simulink model "controlMCUSlugsMKII"  (Simulink 6.6)
settings: Solver=FixedStepDiscrete  StartTime=0.0  StopTime=10.0  FixedStep=0.01  RelTol=1e-3
InitFcn:
  | mcuInit
values from neighbouring files (symbols this model uses):
  T = 0.01    [initGPS.m]    (also in mcuInit.m)
undefined symbols (not defined in the file or in its folder): apSampleTime, bankCommandLimit, baseHeight, bda, bde, bdr, bdt, bICda, bICde, bICdr, bICdt, controlMCUInit, daLimit, deLimit, drLimit, dtLimit, getAccBias, getAccels, getAttitude, getMidLevelCommands, getPassValues, getPidIdx, getWP, getXYZ, gsRead, ISA_g, mda, mde, mdr, mdt, mICda, mICde, mICdr, mICdt, pitchCommandLimit, prepareTelemetry, protParseDecode, protParseDecodeGS, readIpc, send2GS, setCurrentCommands, setDiagnosticFloat, setDiagnosticShort, setNavLat, setNavLong, setNavNav, u1, u2, updateEuler, updateLoad, updatePQR, updatePWM, updatePWM2, y1
libraries: dsPICdrivers x82, simulink x43, SLUGS_Library x27, aerolibconvert2 x3, aerolibutil x3
(part 3 of 5)

== system controlMCUSlugsMKII/Trim Vals/Grab I.C./Convert to Rad2 ==
  IC : Inport  Orientation=down
  Add : Sum  OutScaling=2^-10
  Constant1 : Constant  Value=slopem
  Constant2 : Constant  Value=interceptb
  Data Type Conversion : DataTypeConversion  OutDataTypeMode=single
  Divide : Product  OutScaling=2^-10
  Angle (rad) : Outport
  wires:
  Data Type Conversion/1 -> Angle (rad)/1
  IC/1 -> Divide/1
  Constant2/1 -> Add/2
  Divide/1 -> Add/1
  Add/1 -> Data Type Conversion/1
  Constant1/1 -> Divide/2

== system controlMCUSlugsMKII/Trim Vals/Grab I.C./Convert to Rad3 ==
  IC : Inport  Orientation=down
  Add : Sum  OutScaling=2^-10
  Constant1 : Constant  Value=slopem
  Constant2 : Constant  Value=interceptb
  Data Type Conversion : DataTypeConversion  OutDataTypeMode=single
  Divide : Product  OutScaling=2^-10
  Angle (rad) : Outport
  wires:
  Constant1/1 -> Divide/2
  Add/1 -> Data Type Conversion/1
  Divide/1 -> Add/1
  Constant2/1 -> Add/2
  IC/1 -> Divide/1
  Data Type Conversion/1 -> Angle (rad)/1

== system controlMCUSlugsMKII/Trim Vals/Log  Trims Using PWM High [groundStationDriver.c]/Report Airspeed ==
  Um : Inport  Orientation=down
  Data Type Conversion4 : DataTypeConversion  OutDataTypeMode=uint16  SampleTime=apSampleTime  SaturateOnIntegerOverflow=on
  Gain4 : Gain  Gain=1000
  Update PWM  Commands4 : dsPICdrivers/OTHERS/C Function Call  Tag=dsPIC_dsPIC_CFunctionCall  fctName='updatePWM2'  INPUT_SIZE=1  INPUT1=uint16  INPUT2=uint8  INPUT3=--  OUTPUT_SIZE=1  OUTPUT1=--  SampleTime=-1  InputType=[ 4 2 ]  OutputType=[ ]  FctDeclaration=extern void updatePWM2(uint16_T u1, uint8_T u2);  FctCall=updatePWM2(%u1, %u2);  OrderingInOutPopup=None
  dlf1 : Constant  Value=4  OutDataTypeMode=uint8
  wires:
  Data Type Conversion4/1 -> Update PWM  Commands4/1
  dlf1/1 -> Update PWM  Commands4/2
  Gain4/1 -> Data Type Conversion4/1
  Um/1 -> Gain4/1

== system controlMCUSlugsMKII/Update PWM Commands and Send Telemetry/Generate PWM Signals Based on the Control Type/If  Control Type Is Manual ==
  Pilot (IC) : Inport
  Action Port : ActionPort  ActionType=then
  Demux : Demux
  Gain{,1..3} (4 alike) : Gain  Gain=0.5
  myMux Fun1 : Stateflow chart
  PWM : Outport
  wires:
  Gain/1 -> myMux Fun1/1(u1)
  Gain1/1 -> myMux Fun1/2(u2)
  Gain2/1 -> myMux Fun1/3(u3)
  Gain3/1 -> myMux Fun1/4(u4)
  Demux/1 -> Gain/1
  Demux/2 -> Gain1/1
  Demux/3 -> Gain2/1
  Demux/4 -> Gain3/1
  myMux Fun1/1(y) -> PWM/1
  Pilot (IC)/1 -> Demux/1

== system controlMCUSlugsMKII/Update PWM Commands and Send Telemetry/Generate PWM Signals Based on the Control Type/If  Control Type Is Passthrough ==
  Pilot (IC) : Inport
  Action Port : ActionPort  ActionType=elseif
  Demux : Demux
  Gain{,1..3} (4 alike) : Gain  Gain=0.5
  myMux Fun1 : Stateflow chart
  PWM (abs) : Outport
  wires:
  Gain/1 -> myMux Fun1/1(u1)
  Gain1/1 -> myMux Fun1/2(u2)
  Gain2/1 -> myMux Fun1/3(u3)
  Gain3/1 -> myMux Fun1/4(u4)
  Demux/1 -> Gain/1
  Demux/2 -> Gain1/1
  Demux/3 -> Gain2/1
  Demux/4 -> Gain3/1
  myMux Fun1/1(y) -> PWM (abs)/1
  Pilot (IC)/1 -> Demux/1

== system controlMCUSlugsMKII/Update PWM Commands and Send Telemetry/Generate PWM Signals Based on the Control Type/If  Control Type Is Selective Passthrough ==
  PWM(rad) : Inport
  Pilot (IC) : Inport  Port=2
  Action Port : ActionPort  ActionType=elseif
  Convert to PWM : Subsystem  mask{slopem=mde, interceptb=bde}
      mask prompts: slopem "Slope"; interceptb "Intercept"
  Convert to PWM1 : Subsystem  mask{slopem=mdt, interceptb=bdt}
      mask prompts: slopem "Slope"; interceptb "Intercept"
  Convert to PWM2 : Subsystem  mask{slopem=mda, interceptb=bda}
      mask prompts: slopem "Slope"; interceptb "Intercept"
  Convert to PWM3 : Subsystem  mask{slopem=mdr, interceptb=bdr}
      mask prompts: slopem "Slope"; interceptb "Intercept"
  Demux : Demux  Orientation=down
  Demux1 : Demux
  Demux2 : Demux
  Gain{,1..3} (4 alike) : Gain  Gain=0.5
  Get Pass Switches [navSupport.c] : dsPICdrivers/OTHERS/C Function Call  Tag=dsPIC_dsPIC_CFunctionCall  fctName='getPassValues'  INPUT_SIZE=1  INPUT1=--  INPUT2=--  INPUT3=--  OUTPUT_SIZE=4  OUTPUT1=uint8  SampleTime=.01  InputType=[ ]  OutputType=[ 2 ]  FctDeclaration=extern void getPassValues(uint8_T* y1);  FctCall=getPassValues(*%y1);  OrderingInOutPopup=None
  Switch{,1..3} (4 alike) : Switch  Threshold=0.5
  myMux Fun1 : Stateflow chart
  PWM : Outport
  wires:
  myMux Fun1/1(y) -> PWM/1
  Switch/1 -> myMux Fun1/1(u1)
  Switch1/1 -> myMux Fun1/2(u2)
  Switch2/1 -> myMux Fun1/3(u3)
  Switch3/1 -> myMux Fun1/4(u4)
  Get Pass Switches [navSupport.c]/1 -> Demux/1
  Demux/4 -> Switch/2
  Demux/3 -> Switch1/2
  Demux/2 -> Switch2/2
  Demux/1 -> Switch3/2
  Demux1/1 -> Convert to PWM1/1(" Angle(rad)")
  Demux1/2 -> Convert to PWM2/1(" Angle(rad)")
  Demux1/3 -> Convert to PWM3/1(" Angle(rad)")
  Demux1/4 -> Convert to PWM/1(" Angle(rad)")
  PWM(rad)/1 -> Demux1/1
  Convert to PWM1/1(PWM) -> Switch/3
  Convert to PWM2/1(PWM) -> Switch1/3
  Convert to PWM3/1(PWM) -> Switch2/3
  Convert to PWM/1(PWM) -> Switch3/3
  Demux2/1 -> Gain/1
  Demux2/2 -> Gain1/1
  Demux2/3 -> Gain2/1
  Demux2/4 -> Gain3/1
  Pilot (IC)/1 -> Demux2/1
  Gain/1 -> Switch/1
  Gain1/1 -> Switch1/1
  Gain2/1 -> Switch2/1
  Gain3/1 -> Switch3/1

== system controlMCUSlugsMKII/Update PWM Commands and Send Telemetry/Generate PWM Signals Based on the Control Type/If  Control Type Is Wp Follow  or Inner Cmds ==
  PWM(rad) : Inport
  Action Port : ActionPort  ActionType=elseif
  Convert to PWM : Subsystem  mask{slopem=mde, interceptb=bde}
      mask prompts: slopem "Slope"; interceptb "Intercept"
  Convert to PWM1 : Subsystem  mask{slopem=mdt, interceptb=bdt}
      mask prompts: slopem "Slope"; interceptb "Intercept"
  Convert to PWM2 : Subsystem  mask{slopem=mda, interceptb=bda}
      mask prompts: slopem "Slope"; interceptb "Intercept"
  Convert to PWM3 : Subsystem  mask{slopem=mdr, interceptb=bdr}
      mask prompts: slopem "Slope"; interceptb "Intercept"
  Demux : Demux
  myMux Fun1 : Stateflow chart
  PWM (abs) : Outport
  wires:
  myMux Fun1/1(y) -> PWM (abs)/1
  Convert to PWM1/1(PWM) -> myMux Fun1/1(u1)
  Convert to PWM2/1(PWM) -> myMux Fun1/2(u2)
  Convert to PWM3/1(PWM) -> myMux Fun1/3(u3)
  Convert to PWM/1(PWM) -> myMux Fun1/4(u4)
  Demux/1 -> Convert to PWM1/1(" Angle(rad)")
  Demux/2 -> Convert to PWM2/1(" Angle(rad)")
  Demux/3 -> Convert to PWM3/1(" Angle(rad)")
  Demux/4 -> Convert to PWM/1(" Angle(rad)")
  PWM(rad)/1 -> Demux/1

== system controlMCUSlugsMKII/get Nav Vars/Direction Cosine Matrix to Euler Angles/Subsystem1 ==
  u : Inport
  v : Inport  Port=2
  C Function Call : dsPICdrivers/OTHERS/C Function Call  Tag=dsPIC_dsPIC_CFunctionCall  fctName='myAtan2'  INPUT_SIZE=1  INPUT1=real32  INPUT2=real32  INPUT3=--  OUTPUT_SIZE=1  OUTPUT1=real32  SampleTime=-1  InputType=[ 7 7 ]  OutputType=[ 7 ]  FctDeclaration=extern real32_T myAtan2(real32_T u1, real32_T u2);  FctCall=%y1 = myAtan2(%u1, %u2);  OrderingInOutPopup=None
  atan2(x,y) : Outport
  wires:
  C Function Call/1 -> atan2(x,y)/1
  v/1 -> C Function Call/2
  u/1 -> C Function Call/1

== system controlMCUSlugsMKII/get Nav Vars/Direction Cosine Matrix to Euler Angles/Subsystem2 ==
  u : Inport
  v : Inport  Port=2
  C Function Call : dsPICdrivers/OTHERS/C Function Call  Tag=dsPIC_dsPIC_CFunctionCall  fctName='myAtan2'  INPUT_SIZE=1  INPUT1=real32  INPUT2=real32  INPUT3=--  OUTPUT_SIZE=1  OUTPUT1=real32  SampleTime=-1  InputType=[ 7 7 ]  OutputType=[ 7 ]  FctDeclaration=extern real32_T myAtan2(real32_T u1, real32_T u2);  FctCall=%y1 = myAtan2(%u1, %u2);  OrderingInOutPopup=None
  atan2(x,y) : Outport
  wires:
  u/1 -> C Function Call/1
  v/1 -> C Function Call/2
  C Function Call/1 -> atan2(x,y)/1

== system controlMCUSlugsMKII/get Nav Vars/Direction Cosine Matrix to Euler Angles/Subsystem3 ==
  x : Inport
  C Function Call : dsPICdrivers/OTHERS/C Function Call  Tag=dsPIC_dsPIC_CFunctionCall  fctName='myAsin'  INPUT_SIZE=1  INPUT1=real32  INPUT2=--  INPUT3=--  OUTPUT_SIZE=1  OUTPUT1=real32  SampleTime=-1  InputType=[ 7 ]  OutputType=[ 7 ]  FctDeclaration=extern real32_T myAsin(real32_T u1);  FctCall=%y1 = myAsin(%u1);  OrderingInOutPopup=None
  "[-1,1]" : Saturate  UpperLimit=0.9999  LowerLimit=-0.999
  asin(x) : Outport
  wires:
  C Function Call/1 -> asin(x)/1
  x/1 -> "[-1,1]"/1
  "[-1,1]"/1 -> C Function Call/1

== system controlMCUSlugsMKII/get Nav Vars/Direction Cosine Matrix to Euler Angles/cos(phi)cos(theta) ==
  DCM : Inport
  Demux : Demux  Outputs=9
  Terminator{,1..7} (8 alike) : Terminator
  cos(phi)cos(theta) : Outport
  wires:
  Demux/4 -> Terminator/1
  Demux/3 -> Terminator1/1
  Demux/5 -> Terminator4/1
  Demux/2 -> Terminator3/1
  Demux/1 -> Terminator2/1
  DCM/1 -> Demux/1
  Demux/8 -> Terminator7/1
  Demux/6 -> Terminator5/1
  Demux/7 -> Terminator6/1
  Demux/9 -> cos(phi)cos(theta)/1

== system controlMCUSlugsMKII/get Nav Vars/Direction Cosine Matrix to Euler Angles/cos(psi)cos(theta) ==
  DCM : Inport
  Demux : Demux  Outputs=9
  Terminator{,1..7} (8 alike) : Terminator
  cos(psi)cos(theta) : Outport
  wires:
  Demux/9 -> Terminator2/1
  Demux/7 -> Terminator6/1
  Demux/6 -> Terminator5/1
  Demux/8 -> Terminator7/1
  DCM/1 -> Demux/1
  Demux/1 -> cos(psi)cos(theta)/1
  Demux/2 -> Terminator3/1
  Demux/5 -> Terminator4/1
  Demux/3 -> Terminator1/1
  Demux/4 -> Terminator/1

== system controlMCUSlugsMKII/get Nav Vars/Direction Cosine Matrix to Euler Angles/sin(phi)cos(theta) ==
  DCM : Inport
  Demux : Demux  Outputs=9
  Terminator{,1..7} (8 alike) : Terminator
  sin(phi)cos(theta) : Outport
  wires:
  Demux/9 -> Terminator7/1
  Demux/7 -> Terminator6/1
  Demux/6 -> Terminator5/1
  Demux/8 -> sin(phi)cos(theta)/1
  DCM/1 -> Demux/1
  Demux/1 -> Terminator2/1
  Demux/2 -> Terminator3/1
  Demux/5 -> Terminator4/1
  Demux/3 -> Terminator1/1
  Demux/4 -> Terminator/1

== system controlMCUSlugsMKII/get Nav Vars/Direction Cosine Matrix to Euler Angles/sin(psi)cos(theta) ==
  DCM : Inport
  Demux : Demux  Outputs=9
  Terminator{,1..7} (8 alike) : Terminator
  sin(psi)cos(theta) : Outport
  wires:
  Demux/4 -> sin(psi)cos(theta)/1
  Demux/3 -> Terminator1/1
  Demux/5 -> Terminator4/1
  Demux/2 -> Terminator3/1
  Demux/1 -> Terminator2/1
  DCM/1 -> Demux/1
  Demux/8 -> Terminator/1
  Demux/6 -> Terminator5/1
  Demux/7 -> Terminator6/1
  Demux/9 -> Terminator7/1

== system controlMCUSlugsMKII/get Nav Vars/Direction Cosine Matrix to Euler Angles/sin(theta) ==
  DCM : Inport
  Demux : Demux  Outputs=9
  Gain2 : Gain  Gain=-1  SaturateOnIntegerOverflow=on
  Terminator{,1..5,7..8} (8 alike) : Terminator
  sin(theta) : Outport
  wires:
  Gain2/1 -> sin(theta)/1
  Demux/4 -> Terminator/1
  Demux/3 -> Terminator1/1
  Demux/5 -> Terminator4/1
  Demux/2 -> Terminator3/1
  Demux/1 -> Terminator2/1
  DCM/1 -> Demux/1
  Demux/8 -> Terminator8/1
  Demux/6 -> Terminator5/1
  Demux/7 -> Gain2/1
  Demux/9 -> Terminator7/1

== system controlMCUSlugsMKII/get Nav Vars/Euler Angles to  Direction Cosine Matrix1/A11 ==
  sin_cos : Inport
  Demux : Demux  Outputs=6
  Terminator{,1..3} (4 alike) : Terminator
  u(5)*u(6) : Product  RndMeth=Zero
  A11 : Outport
  wires:
  Demux/6 -> u(5)*u(6)/2
  u(5)*u(6)/1 -> A11/1
  sin_cos/1 -> Demux/1
  Demux/1 -> Terminator2/1
  Demux/2 -> Terminator3/1
  Demux/5 -> u(5)*u(6)/1
  Demux/3 -> Terminator1/1
  Demux/4 -> Terminator/1

== system controlMCUSlugsMKII/get Nav Vars/Euler Angles to  Direction Cosine Matrix1/A12 ==
  sin_cos : Inport
  Demux : Demux  Outputs=6
  Terminator{,1..3} (4 alike) : Terminator
  u(3)*u(5) : Product  RndMeth=Zero
  A12 : Outport
  wires:
  Demux/4 -> Terminator/1
  Demux/3 -> u(3)*u(5)/1
  Demux/5 -> u(3)*u(5)/2
  Demux/2 -> Terminator3/1
  Demux/1 -> Terminator2/1
  sin_cos/1 -> Demux/1
  u(3)*u(5)/1 -> A12/1
  Demux/6 -> Terminator1/1

== system controlMCUSlugsMKII/get Nav Vars/Euler Angles to  Direction Cosine Matrix1/A13 ==
  sin_cos : Inport
  Demux : Demux  Outputs=6
  Gain2 : Gain  Gain=-1  SaturateOnIntegerOverflow=on
  Terminator{,1..4} (5 alike) : Terminator
  A13 : Outport
  wires:
  Demux/6 -> Terminator1/1
  sin_cos/1 -> Demux/1
  Demux/1 -> Terminator2/1
  Demux/2 -> Gain2/1
  Demux/5 -> Terminator4/1
  Demux/3 -> Terminator3/1
  Demux/4 -> Terminator/1
  Gain2/1 -> A13/1

== system controlMCUSlugsMKII/get Nav Vars/Euler Angles to  Direction Cosine Matrix1/A21 ==
  sin_cos : Inport
  Demux : Demux  Outputs=6
  Sum : Sum  Inputs=|+-
  Terminator : Terminator
  u(3)*u(4) : Product  RndMeth=Zero
  u(6)*u(1)*u(2) : Product  Inputs=3  RndMeth=Zero
  A21 : Outport
  wires:
  Sum/1 -> A21/1
  u(3)*u(4)/1 -> Sum/2
  u(6)*u(1)*u(2)/1 -> Sum/1
  sin_cos/1 -> Demux/1
  Demux/1 -> u(6)*u(1)*u(2)/2
  Demux/2 -> u(6)*u(1)*u(2)/3
  Demux/5 -> Terminator/1
  Demux/6 -> u(6)*u(1)*u(2)/1
  Demux/3 -> u(3)*u(4)/1
  Demux/4 -> u(3)*u(4)/2

== system controlMCUSlugsMKII/get Nav Vars/Euler Angles to  Direction Cosine Matrix1/A22 ==
  sin_cos : Inport
  Demux : Demux  Outputs=6
  Sum : Sum  Inputs=|++
  Terminator : Terminator
  u(1)*u(2)*u(3) : Product  Inputs=3  RndMeth=Zero
  u(4)*u(6) : Product  RndMeth=Zero
  A22 : Outport
  wires:
  Demux/4 -> u(4)*u(6)/1
  Demux/3 -> u(1)*u(2)*u(3)/3
  Demux/5 -> Terminator/1
  Demux/2 -> u(1)*u(2)*u(3)/2
  Demux/1 -> u(1)*u(2)*u(3)/1
  sin_cos/1 -> Demux/1
  u(1)*u(2)*u(3)/1 -> Sum/1
  u(4)*u(6)/1 -> Sum/2
  Sum/1 -> A22/1
  Demux/6 -> u(4)*u(6)/2

== system controlMCUSlugsMKII/get Nav Vars/Euler Angles to  Direction Cosine Matrix1/A23 ==
  sin_cos : Inport
  Demux : Demux  Outputs=6
  Terminator{,1..3} (4 alike) : Terminator
  u(1)*u(3) : Product  RndMeth=Zero
  A23 : Outport
  wires:
  Demux/6 -> Terminator1/1
  u(1)*u(3)/1 -> A23/1
  sin_cos/1 -> Demux/1
  Demux/1 -> u(1)*u(3)/1
  Demux/2 -> Terminator3/1
  Demux/5 -> u(1)*u(3)/2
  Demux/3 -> Terminator2/1
  Demux/4 -> Terminator/1

== system controlMCUSlugsMKII/get Nav Vars/Euler Angles to  Direction Cosine Matrix1/A31 ==
  sin_cos : Inport
  Demux : Demux  Outputs=6
  Sum : Sum  Inputs=|++
  Terminator : Terminator
  u(1)*u(3) : Product  RndMeth=Zero
  u(2)*u(4)*u(6) : Product  Inputs=3  RndMeth=Zero
  A31 : Outport
  wires:
  Demux/4 -> u(2)*u(4)*u(6)/2
  Demux/3 -> u(1)*u(3)/2
  Demux/5 -> Terminator/1
  Demux/2 -> u(2)*u(4)*u(6)/1
  Demux/1 -> u(1)*u(3)/1
  sin_cos/1 -> Demux/1
  u(2)*u(4)*u(6)/1 -> Sum/2
  Sum/1 -> A31/1
  Demux/6 -> u(2)*u(4)*u(6)/3
  u(1)*u(3)/1 -> Sum/1

== system controlMCUSlugsMKII/get Nav Vars/Euler Angles to  Direction Cosine Matrix1/A32 ==
  sin_cos : Inport
  Demux : Demux  Outputs=6
  Sum : Sum  Inputs=|+-
  Terminator : Terminator
  u(1)*u(6) : Product  RndMeth=Zero
  u(2)*u(3)*u(4) : Product  Inputs=3  RndMeth=Zero
  A32 : Outport
  wires:
  Demux/6 -> u(1)*u(6)/1
  Sum/1 -> A32/1
  u(1)*u(6)/1 -> Sum/2
  u(2)*u(3)*u(4)/1 -> Sum/1
  sin_cos/1 -> Demux/1
  Demux/1 -> u(1)*u(6)/2
  Demux/2 -> u(2)*u(3)*u(4)/1
  Demux/5 -> Terminator/1
  Demux/3 -> u(2)*u(3)*u(4)/2
  Demux/4 -> u(2)*u(3)*u(4)/3

== system controlMCUSlugsMKII/get Nav Vars/Euler Angles to  Direction Cosine Matrix1/A33 ==
  sin_cos : Inport
  Demux : Demux  Outputs=6
  Terminator{,1..3} (4 alike) : Terminator
  u(4)*u(5) : Product  RndMeth=Zero
  A33 : Outport
  wires:
  Demux/4 -> u(4)*u(5)/1
  Demux/3 -> Terminator1/1
  Demux/5 -> u(4)*u(5)/2
  Demux/2 -> Terminator3/1
  Demux/1 -> Terminator2/1
  sin_cos/1 -> Demux/1
  u(4)*u(5)/1 -> A33/1
  Demux/6 -> Terminator/1

== system controlMCUSlugsMKII/get Nav Vars/Euler Angles to  Direction Cosine Matrix1/Create Transformation Matrix ==
  M11 : Inport
  M12 : Inport  Port=2
  M13 : Inport  Port=3
  M21 : Inport  Port=4
  M22 : Inport  Port=5
  M23 : Inport  Port=6
  M31 : Inport  Port=7
  M32 : Inport  Port=8
  M33 : Inport  Port=9
  Reshape (9) to [3x3] column-major : Reshape  OutputDimensionality=Customize  OutputDimensions=[3,3]
  myMux Fun1 : Stateflow chart
  Matrix : Outport
  wires:
  myMux Fun1/1(y) -> Reshape (9) to [3x3] column-major/1
  M11/1 -> myMux Fun1/1(u1)
  M21/1 -> myMux Fun1/2(u2)
  M31/1 -> myMux Fun1/3(u3)
  M12/1 -> myMux Fun1/4(u4)
  M22/1 -> myMux Fun1/5(u5)
  Reshape (9) to [3x3] column-major/1 -> Matrix/1
  M32/1 -> myMux Fun1/6(u6)
  M13/1 -> myMux Fun1/7(u7)
  M23/1 -> myMux Fun1/8(u8)
  M33/1 -> myMux Fun1/9(u9)

== system controlMCUSlugsMKII/get Nav Vars/Euler Angles to  Direction Cosine Matrix1/Subsystem5 ==
  u : Inport
  C Function Call : dsPICdrivers/OTHERS/C Function Call  Tag=dsPIC_dsPIC_CFunctionCall  fctName='mySin'  INPUT_SIZE=1  INPUT1=real32  INPUT2=--  INPUT3=--  OUTPUT_SIZE=1  OUTPUT1=real32  SampleTime=-1  InputType=[ 7 ]  OutputType=[ 7 ]  FctDeclaration=extern real32_T mySin(real32_T u1);  FctCall=%y1 = mySin(%u1);  OrderingInOutPopup=None
  C Function Call1 : dsPICdrivers/OTHERS/C Function Call  Tag=dsPIC_dsPIC_CFunctionCall  fctName='myCos'  INPUT_SIZE=1  INPUT1=real32  INPUT2=--  INPUT3=--  OUTPUT_SIZE=1  OUTPUT1=real32  SampleTime=-1  InputType=[ 7 ]  OutputType=[ 7 ]  FctDeclaration=extern real32_T myCos(real32_T u1);  FctCall=%y1 = myCos(%u1);  OrderingInOutPopup=None
  C Function Call2 : dsPICdrivers/OTHERS/C Function Call  Tag=dsPIC_dsPIC_CFunctionCall  fctName='mySin'  INPUT_SIZE=1  INPUT1=real32  INPUT2=--  INPUT3=--  OUTPUT_SIZE=1  OUTPUT1=real32  SampleTime=-1  InputType=[ 7 ]  OutputType=[ 7 ]  FctDeclaration=extern real32_T mySin(real32_T u1);  FctCall=%y1 = mySin(%u1);  OrderingInOutPopup=None
  C Function Call3 : dsPICdrivers/OTHERS/C Function Call  Tag=dsPIC_dsPIC_CFunctionCall  fctName='mySin'  INPUT_SIZE=1  INPUT1=real32  INPUT2=--  INPUT3=--  OUTPUT_SIZE=1  OUTPUT1=real32  SampleTime=-1  InputType=[ 7 ]  OutputType=[ 7 ]  FctDeclaration=extern real32_T mySin(real32_T u1);  FctCall=%y1 = mySin(%u1);  OrderingInOutPopup=None
  C Function Call4 : dsPICdrivers/OTHERS/C Function Call  Tag=dsPIC_dsPIC_CFunctionCall  fctName='myCos'  INPUT_SIZE=1  INPUT1=real32  INPUT2=--  INPUT3=--  OUTPUT_SIZE=1  OUTPUT1=real32  SampleTime=-1  InputType=[ 7 ]  OutputType=[ 7 ]  FctDeclaration=extern real32_T myCos(real32_T u1);  FctCall=%y1 = myCos(%u1);  OrderingInOutPopup=None
  C Function Call5 : dsPICdrivers/OTHERS/C Function Call  Tag=dsPIC_dsPIC_CFunctionCall  fctName='myCos'  INPUT_SIZE=1  INPUT1=real32  INPUT2=--  INPUT3=--  OUTPUT_SIZE=1  OUTPUT1=real32  SampleTime=-1  InputType=[ 7 ]  OutputType=[ 7 ]  FctDeclaration=extern real32_T myCos(real32_T u1);  FctCall=%y1 = myCos(%u1);  OrderingInOutPopup=None
  Demux : Demux  Outputs=3
  Demux1 : Demux  Outputs=3
  Environment Controller : simulink/Signal Routing/Environment Controller  SystemSampleTime=-1
  Environment Controller1 : simulink/Signal Routing/Environment Controller  SystemSampleTime=-1
  SinCos1 : aerolibutil/SinCos  SystemSampleTime=-1
  myMux Fun1 : Stateflow chart
  myMux Fun2 : Stateflow chart
  sin(u) : Outport
  cos(u) : Outport  Port=2
  wires:
  Environment Controller/1 -> sin(u)/1
  SinCos1/1 -> Environment Controller/1
  u/1 -> SinCos1/1, Demux/1, Demux1/1
  Environment Controller1/1 -> cos(u)/1
  SinCos1/2 -> Environment Controller1/1
  C Function Call/1 -> myMux Fun1/1(u1)
  C Function Call2/1 -> myMux Fun1/2(u2)
  C Function Call3/1 -> myMux Fun1/3(u3)
  C Function Call1/1 -> myMux Fun2/1(u1)
  C Function Call4/1 -> myMux Fun2/2(u2)
  C Function Call5/1 -> myMux Fun2/3(u3)
  Demux/1 -> C Function Call/1
  Demux/2 -> C Function Call2/1
  Demux/3 -> C Function Call3/1
  Demux1/1 -> C Function Call1/1
  Demux1/2 -> C Function Call4/1
  Demux1/3 -> C Function Call5/1
  myMux Fun1/1(y) -> Environment Controller/2
  myMux Fun2/1(y) -> Environment Controller1/2

== system controlMCUSlugsMKII/get Nav Vars/Euler Angles to  Direction Cosine Matrix2/A11 ==
  sin_cos : Inport
  Demux : Demux  Outputs=6
  Terminator{,1..3} (4 alike) : Terminator
  u(5)*u(6) : Product  RndMeth=Zero
  A11 : Outport
  wires:
  Demux/4 -> Terminator/1
  Demux/3 -> Terminator1/1
  Demux/5 -> u(5)*u(6)/1
  Demux/2 -> Terminator3/1
  Demux/1 -> Terminator2/1
  sin_cos/1 -> Demux/1
  u(5)*u(6)/1 -> A11/1
  Demux/6 -> u(5)*u(6)/2

== system controlMCUSlugsMKII/get Nav Vars/Euler Angles to  Direction Cosine Matrix2/A12 ==
  sin_cos : Inport
  Demux : Demux  Outputs=6
  Terminator{,1..3} (4 alike) : Terminator
  u(3)*u(5) : Product  RndMeth=Zero
  A12 : Outport
  wires:
  Demux/6 -> Terminator1/1
  u(3)*u(5)/1 -> A12/1
  sin_cos/1 -> Demux/1
  Demux/1 -> Terminator2/1
  Demux/2 -> Terminator3/1
  Demux/5 -> u(3)*u(5)/2
  Demux/3 -> u(3)*u(5)/1
  Demux/4 -> Terminator/1

== system controlMCUSlugsMKII/get Nav Vars/Euler Angles to  Direction Cosine Matrix2/A13 ==
  sin_cos : Inport
  Demux : Demux  Outputs=6
  Gain2 : Gain  Gain=-1  SaturateOnIntegerOverflow=on
  Terminator{,1..4} (5 alike) : Terminator
  A13 : Outport
  wires:
  Gain2/1 -> A13/1
  Demux/4 -> Terminator/1
  Demux/3 -> Terminator3/1
  Demux/5 -> Terminator4/1
  Demux/2 -> Gain2/1
  Demux/1 -> Terminator2/1
  sin_cos/1 -> Demux/1
  Demux/6 -> Terminator1/1

== system controlMCUSlugsMKII/get Nav Vars/Euler Angles to  Direction Cosine Matrix2/A21 ==
  sin_cos : Inport
  Demux : Demux  Outputs=6
  Sum : Sum  Inputs=|+-
  Terminator : Terminator
  u(3)*u(4) : Product  RndMeth=Zero
  u(6)*u(1)*u(2) : Product  Inputs=3  RndMeth=Zero
  A21 : Outport
  wires:
  Demux/4 -> u(3)*u(4)/2
  Demux/3 -> u(3)*u(4)/1
  Demux/6 -> u(6)*u(1)*u(2)/1
  Demux/5 -> Terminator/1
  Demux/2 -> u(6)*u(1)*u(2)/3
  Demux/1 -> u(6)*u(1)*u(2)/2
  sin_cos/1 -> Demux/1
  u(6)*u(1)*u(2)/1 -> Sum/1
  u(3)*u(4)/1 -> Sum/2
  Sum/1 -> A21/1

== system controlMCUSlugsMKII/get Nav Vars/Euler Angles to  Direction Cosine Matrix2/A22 ==
  sin_cos : Inport
  Demux : Demux  Outputs=6
  Sum : Sum  Inputs=|++
  Terminator : Terminator
  u(1)*u(2)*u(3) : Product  Inputs=3  RndMeth=Zero
  u(4)*u(6) : Product  RndMeth=Zero
  A22 : Outport
  wires:
  Demux/6 -> u(4)*u(6)/2
  Sum/1 -> A22/1
  u(4)*u(6)/1 -> Sum/2
  u(1)*u(2)*u(3)/1 -> Sum/1
  sin_cos/1 -> Demux/1
  Demux/1 -> u(1)*u(2)*u(3)/1
  Demux/2 -> u(1)*u(2)*u(3)/2
  Demux/5 -> Terminator/1
  Demux/3 -> u(1)*u(2)*u(3)/3
  Demux/4 -> u(4)*u(6)/1

== system controlMCUSlugsMKII/get Nav Vars/Euler Angles to  Direction Cosine Matrix2/A23 ==
  sin_cos : Inport
  Demux : Demux  Outputs=6
  Terminator{,1..3} (4 alike) : Terminator
  u(1)*u(3) : Product  RndMeth=Zero
  A23 : Outport
  wires:
  Demux/4 -> Terminator/1
  Demux/3 -> Terminator2/1
  Demux/5 -> u(1)*u(3)/2
  Demux/2 -> Terminator3/1
  Demux/1 -> u(1)*u(3)/1
  sin_cos/1 -> Demux/1
  u(1)*u(3)/1 -> A23/1
  Demux/6 -> Terminator1/1

== system controlMCUSlugsMKII/get Nav Vars/Euler Angles to  Direction Cosine Matrix2/A31 ==
  sin_cos : Inport
  Demux : Demux  Outputs=6
  Sum : Sum  Inputs=|++
  Terminator : Terminator
  u(1)*u(3) : Product  RndMeth=Zero
  u(2)*u(4)*u(6) : Product  Inputs=3  RndMeth=Zero
  A31 : Outport
  wires:
  u(1)*u(3)/1 -> Sum/1
  Demux/6 -> u(2)*u(4)*u(6)/3
  Sum/1 -> A31/1
  u(2)*u(4)*u(6)/1 -> Sum/2
  sin_cos/1 -> Demux/1
  Demux/1 -> u(1)*u(3)/1
  Demux/2 -> u(2)*u(4)*u(6)/1
  Demux/5 -> Terminator/1
  Demux/3 -> u(1)*u(3)/2
  Demux/4 -> u(2)*u(4)*u(6)/2

== system controlMCUSlugsMKII/get Nav Vars/Euler Angles to  Direction Cosine Matrix2/A32 ==
  sin_cos : Inport
  Demux : Demux  Outputs=6
  Sum : Sum  Inputs=|+-
  Terminator : Terminator
  u(1)*u(6) : Product  RndMeth=Zero
  u(2)*u(3)*u(4) : Product  Inputs=3  RndMeth=Zero
  A32 : Outport
  wires:
  Demux/4 -> u(2)*u(3)*u(4)/3
  Demux/3 -> u(2)*u(3)*u(4)/2
  Demux/5 -> Terminator/1
  Demux/2 -> u(2)*u(3)*u(4)/1
  Demux/1 -> u(1)*u(6)/2
  sin_cos/1 -> Demux/1
  u(2)*u(3)*u(4)/1 -> Sum/1
  u(1)*u(6)/1 -> Sum/2
  Sum/1 -> A32/1
  Demux/6 -> u(1)*u(6)/1

== system controlMCUSlugsMKII/get Nav Vars/Euler Angles to  Direction Cosine Matrix2/A33 ==
  sin_cos : Inport
  Demux : Demux  Outputs=6
  Terminator{,1..3} (4 alike) : Terminator
  u(4)*u(5) : Product  RndMeth=Zero
  A33 : Outport
  wires:
  Demux/6 -> Terminator/1
  u(4)*u(5)/1 -> A33/1
  sin_cos/1 -> Demux/1
  Demux/1 -> Terminator2/1
  Demux/2 -> Terminator3/1
  Demux/5 -> u(4)*u(5)/2
  Demux/3 -> Terminator1/1
  Demux/4 -> u(4)*u(5)/1

== system controlMCUSlugsMKII/get Nav Vars/Euler Angles to  Direction Cosine Matrix2/Create Transformation Matrix ==
  M11 : Inport
  M12 : Inport  Port=2
  M13 : Inport  Port=3
  M21 : Inport  Port=4
  M22 : Inport  Port=5
  M23 : Inport  Port=6
  M31 : Inport  Port=7
  M32 : Inport  Port=8
  M33 : Inport  Port=9
  Reshape (9) to [3x3] column-major : Reshape  OutputDimensionality=Customize  OutputDimensions=[3,3]
  myMux Fun1 : Stateflow chart
  Matrix : Outport
  wires:
  M33/1 -> myMux Fun1/9(u9)
  M23/1 -> myMux Fun1/8(u8)
  M13/1 -> myMux Fun1/7(u7)
  M32/1 -> myMux Fun1/6(u6)
  Reshape (9) to [3x3] column-major/1 -> Matrix/1
  M22/1 -> myMux Fun1/5(u5)
  M12/1 -> myMux Fun1/4(u4)
  M31/1 -> myMux Fun1/3(u3)
  M21/1 -> myMux Fun1/2(u2)
  M11/1 -> myMux Fun1/1(u1)
  myMux Fun1/1(y) -> Reshape (9) to [3x3] column-major/1

== system controlMCUSlugsMKII/get Nav Vars/Euler Angles to  Direction Cosine Matrix2/Subsystem5 ==
  u : Inport
  C Function Call : dsPICdrivers/OTHERS/C Function Call  Tag=dsPIC_dsPIC_CFunctionCall  fctName='mySin'  INPUT_SIZE=1  INPUT1=real32  INPUT2=--  INPUT3=--  OUTPUT_SIZE=1  OUTPUT1=real32  SampleTime=-1  InputType=[ 7 ]  OutputType=[ 7 ]  FctDeclaration=extern real32_T mySin(real32_T u1);  FctCall=%y1 = mySin(%u1);  OrderingInOutPopup=None
  C Function Call1 : dsPICdrivers/OTHERS/C Function Call  Tag=dsPIC_dsPIC_CFunctionCall  fctName='myCos'  INPUT_SIZE=1  INPUT1=real32  INPUT2=--  INPUT3=--  OUTPUT_SIZE=1  OUTPUT1=real32  SampleTime=-1  InputType=[ 7 ]  OutputType=[ 7 ]  FctDeclaration=extern real32_T myCos(real32_T u1);  FctCall=%y1 = myCos(%u1);  OrderingInOutPopup=None
  C Function Call2 : dsPICdrivers/OTHERS/C Function Call  Tag=dsPIC_dsPIC_CFunctionCall  fctName='mySin'  INPUT_SIZE=1  INPUT1=real32  INPUT2=--  INPUT3=--  OUTPUT_SIZE=1  OUTPUT1=real32  SampleTime=-1  InputType=[ 7 ]  OutputType=[ 7 ]  FctDeclaration=extern real32_T mySin(real32_T u1);  FctCall=%y1 = mySin(%u1);  OrderingInOutPopup=None
  C Function Call3 : dsPICdrivers/OTHERS/C Function Call  Tag=dsPIC_dsPIC_CFunctionCall  fctName='mySin'  INPUT_SIZE=1  INPUT1=real32  INPUT2=--  INPUT3=--  OUTPUT_SIZE=1  OUTPUT1=real32  SampleTime=-1  InputType=[ 7 ]  OutputType=[ 7 ]  FctDeclaration=extern real32_T mySin(real32_T u1);  FctCall=%y1 = mySin(%u1);  OrderingInOutPopup=None
  C Function Call4 : dsPICdrivers/OTHERS/C Function Call  Tag=dsPIC_dsPIC_CFunctionCall  fctName='myCos'  INPUT_SIZE=1  INPUT1=real32  INPUT2=--  INPUT3=--  OUTPUT_SIZE=1  OUTPUT1=real32  SampleTime=-1  InputType=[ 7 ]  OutputType=[ 7 ]  FctDeclaration=extern real32_T myCos(real32_T u1);  FctCall=%y1 = myCos(%u1);  OrderingInOutPopup=None
  C Function Call5 : dsPICdrivers/OTHERS/C Function Call  Tag=dsPIC_dsPIC_CFunctionCall  fctName='myCos'  INPUT_SIZE=1  INPUT1=real32  INPUT2=--  INPUT3=--  OUTPUT_SIZE=1  OUTPUT1=real32  SampleTime=-1  InputType=[ 7 ]  OutputType=[ 7 ]  FctDeclaration=extern real32_T myCos(real32_T u1);  FctCall=%y1 = myCos(%u1);  OrderingInOutPopup=None
  Demux : Demux  Outputs=3
  Demux1 : Demux  Outputs=3
  Environment Controller : simulink/Signal Routing/Environment Controller  SystemSampleTime=-1
  Environment Controller1 : simulink/Signal Routing/Environment Controller  SystemSampleTime=-1
  SinCos1 : aerolibutil/SinCos  SystemSampleTime=-1
  myMux Fun1 : Stateflow chart
  myMux Fun2 : Stateflow chart
  sin(u) : Outport
  cos(u) : Outport  Port=2
  wires:
  myMux Fun2/1(y) -> Environment Controller1/2
  myMux Fun1/1(y) -> Environment Controller/2
  Demux1/3 -> C Function Call5/1
  Demux1/2 -> C Function Call4/1
  Demux1/1 -> C Function Call1/1
  Demux/3 -> C Function Call3/1
  Demux/2 -> C Function Call2/1
  Demux/1 -> C Function Call/1
  C Function Call5/1 -> myMux Fun2/3(u3)
  C Function Call4/1 -> myMux Fun2/2(u2)
  C Function Call1/1 -> myMux Fun2/1(u1)
  C Function Call3/1 -> myMux Fun1/3(u3)
  C Function Call2/1 -> myMux Fun1/2(u2)
  C Function Call/1 -> myMux Fun1/1(u1)
  SinCos1/2 -> Environment Controller1/1
  Environment Controller1/1 -> cos(u)/1
  u/1 -> Demux1/1, Demux/1, SinCos1/1
  SinCos1/1 -> Environment Controller/1
  Environment Controller/1 -> sin(u)/1

== system controlMCUSlugsMKII/Inner Loop/ Navigation/L1 Output Feedback Controller With  Projection Operator/Control  Law/Compute Coef ==
  a : Inport
  Enable : EnablePort
  -T : Gain  Gain=-apSampleTime  SampleTime=apSampleTime
  1-c : Sum  Inputs=-+  OutDataTypeMode=single  OutScaling=2^-10  SampleTime=apSampleTime
  Constant : Constant
  Subsystem11 : Subsystem  AncestorBlock=SLUGS_Library/Subsystem11
  b : Outport
  c : Outport  Port=2
  wires:
  -T/1 -> Subsystem11/1(u)
  Subsystem11/1(exp(u)) -> 1-c/1, c/1  "c"
  Constant/1 -> 1-c/2
  1-c/1 -> b/1
  a/1 -> -T/1

== system controlMCUSlugsMKII/Inner Loop/ Navigation/L1 Output Feedback Controller With  Projection Operator/Control  Law/Detect Change ==
  Data : Inport
  Abs1 : Abs  SampleTime=apSampleTime
  Difference1 : simulink/Discrete/Difference  SystemSampleTime=-1  ICPrevInput=0.0  OutDataType=sfix(16)  OutScaling=2^-10  DoSatur=off
  Saturation1 : Saturate  UpperLimit=1  LowerLimit=0  SampleTime=apSampleTime
  change? : Outport
  wires:
  Difference1/1 -> Abs1/1
  Abs1/1 -> Saturation1/1
  Data/1 -> Difference1/1
  Saturation1/1 -> change?/1

== system controlMCUSlugsMKII/Inner Loop/ Navigation/L1 Output Feedback Controller With  Projection Operator/Projection Operator/Enabled Subsystem ==
  In1 : Inport
  Enable : EnablePort
  Out1 : Outport
  wires:
  In1/1 -> Out1/1

== system controlMCUSlugsMKII/Inner Loop/ Navigation/L1 Output Feedback Controller With  Projection Operator/Projection Operator/Enabled Subsystem1 ==
  y : Inport
  f_the : Inport  Port=2
  grad : Inport  Port=3
  Enable : EnablePort
  Constant : Constant  OutDataTypeMode=single
  Divide1 : Product  OutDataTypeMode=single  OutScaling=2^-10
  Divide2 : Product  OutDataTypeMode=single  OutScaling=2^-10
  Sign : Signum
  Subtract : Sum  Inputs=+-  OutDataTypeMode=single  OutScaling=2^-10
  Out1 : Outport
  wires:
  Divide1/1 -> Subtract/2
  grad/1 -> Sign/1
  Sign/1 -> Divide1/2
  Constant/1 -> Subtract/1
  f_the/1 -> Divide1/1
  Subtract/1 -> Divide2/2
  y/1 -> Divide2/1
  Divide2/1 -> Out1/1

== system controlMCUSlugsMKII/Inner Loop/ Navigation/L1 Output Feedback Controller With  Projection Operator/Projection Operator/F(theta) ==
  Theta Max : Inport
  Eps 0 : Inport  Port=2
  Theta : Inport  Port=3
  Constant : Constant  Value=2  OutDataTypeMode=single
  Divide : Product  OutDataTypeMode=single  OutScaling=2^-10
  Divide1 : Product  OutDataTypeMode=single  OutScaling=2^-10
  Divide2 : Product  OutDataTypeMode=single  OutScaling=2^-10
  Divide3 : Product  Inputs=*/  OutDataTypeMode=single  OutScaling=2^-10
  Divide4 : Product  Inputs=/**  OutDataTypeMode=single  OutScaling=2^-10
  Subtract : Sum  Inputs=+-  OutDataTypeMode=single  OutScaling=2^-10
  "Theta " : InportShadow  Port=3  LatchByCopyingInsideSignal=off
  f_theta : Outport
  dif_f_theta : Outport  Port=2
  wires:
  Theta/1 -> Divide/1, Divide/2
  Theta Max/1 -> Divide1/2, Divide1/1
  Divide/1 -> Subtract/1
  Divide1/1 -> Subtract/2, Divide2/1
  Eps 0/1 -> Divide2/2
  Subtract/1 -> Divide3/1
  Divide2/1 -> Divide3/2, Divide4/1
  Divide3/1 -> f_theta/1
  Constant/1 -> Divide4/3
  "Theta "/1 -> Divide4/2
  Divide4/1 -> dif_f_theta/1

== system controlMCUSlugsMKII/Inner Loop/ Navigation/L1 Output Feedback Controller With  Projection Operator/State Predictor/Compute Coef ==
  a : Inport
  Enable : EnablePort
  -T : Gain  Gain=-apSampleTime  SampleTime=apSampleTime
  1-c : Sum  Inputs=-+  OutDataTypeMode=single  OutScaling=2^-10
  Constant : Constant
  Subsystem11 : Subsystem  AncestorBlock=SLUGS_Library/Subsystem11
  b : Outport
  c : Outport  Port=2
  wires:
  a/1 -> -T/1
  1-c/1 -> b/1
  Constant/1 -> 1-c/2
  Subsystem11/1(exp(u)) -> c/1, 1-c/1  "c"
  -T/1 -> Subsystem11/1(u)

== system controlMCUSlugsMKII/Inner Loop/ Navigation/L1 Output Feedback Controller With  Projection Operator/State Predictor/Detect Change ==
  Data : Inport
  Abs1 : Abs  SampleTime=apSampleTime
  Difference1 : simulink/Discrete/Difference  SystemSampleTime=-1  ICPrevInput=0.0  OutDataType=sfix(16)  OutScaling=2^-10  DoSatur=off
  Saturation1 : Saturate  UpperLimit=1  LowerLimit=0  SampleTime=apSampleTime
  change? : Outport
  wires:
  Saturation1/1 -> change?/1
  Data/1 -> Difference1/1
  Abs1/1 -> Saturation1/1
  Difference1/1 -> Abs1/1

== system controlMCUSlugsMKII/Inner Loop/ Navigation/Lateral Channel/Sideslip Compensation/Bank to Psi Dot ==
  phi_c : Inport
  U_m : Inport  Port=2
  Constant1 : Constant  Value=9.80665  OutDataTypeMode=single
  Divide : Product  Inputs=/*  OutDataTypeMode=single  OutScaling=2^-10  SampleTime=apSampleTime
  Divide1 : Product  OutDataTypeMode=single  OutScaling=2^-10  SampleTime=apSampleTime
  Subsystem8 : SLUGS_Library/Subsystem8  SystemSampleTime=-1
  bank Limit : Saturate  UpperLimit=bankCommandLimit  LowerLimit=-bankCommandLimit
  negprotect : Stateflow chart
  psi_dot_c : Outport
  wires:
  U_m/1 -> negprotect/1(val)
  Constant1/1 -> Divide/2
  Divide1/1 -> psi_dot_c/1
  Subsystem8/1 -> Divide1/1
  phi_c/1 -> bank Limit/1
  Divide/1 -> Divide1/2
  negprotect/1(zpVal) -> Divide/1
  bank Limit/1 -> Subsystem8/1

== system controlMCUSlugsMKII/Inner Loop/ Navigation/Lateral Channel/Sideslip Compensation/Low Pass ==
  a : Inport
  u : Inport  Port=2
  Compute Coef : Subsystem
  Detect Change : Subsystem
  Divide : Product  OutScaling=2^-10  SampleTime=apSampleTime
  Divide1 : Product  OutScaling=2^-10  SampleTime=apSampleTime
  IC : InitialCondition
  Integer Delay : simulink/Discrete/Integer Delay  vinit=0.0  samptime=apSampleTime  NumDelays=1
  Integer Delay1 : simulink/Discrete/Integer Delay  Orientation=left  vinit=0.0  samptime=apSampleTime  NumDelays=1
  Subtract : Sum  OutScaling=2^-10  SampleTime=apSampleTime
  y : Outport
  wires:
  Integer Delay1/1 -> Divide1/2
  u/1 -> Integer Delay/1
  IC/1 -> Compute Coef/Enable
  Subtract/1 -> Integer Delay1/1, y/1
  Divide1/1 -> Subtract/2
  Divide/1 -> Subtract/1
  Integer Delay/1 -> Divide/2
  Detect Change/1(change?) -> IC/1
  Compute Coef/2(c) -> Divide1/1
  Compute Coef/1(b) -> Divide/1
  a/1 -> Detect Change/1(Data), Compute Coef/1(a)

== system controlMCUSlugsMKII/Inner Loop/ Navigation/Lateral Channel/Sideslip Compensation/psi_dot to Bank ==
  psi_dot_c : Inport
  U_m : Inport  Port=2
  Constant1 : Constant  Value=9.80665  OutDataTypeMode=single
  Divide : Product  Inputs=**/  OutScaling=2^-10  SampleTime=apSampleTime
  Subsystem2 : SLUGS_Library/Subsystem2  SystemSampleTime=-1
  phi_c : Outport
  wires:
  psi_dot_c/1 -> Divide/1
  U_m/1 -> Divide/2
  Constant1/1 -> Divide/3
  Subsystem2/1 -> phi_c/1
  Divide/1 -> Subsystem2/1

== system controlMCUSlugsMKII/Inner Loop/ Navigation/Longitudinal Channel/Air Density from Height/Subsystem ==
  u : Inport
  v : Inport  Port=2
  C Function Call : dsPICdrivers/OTHERS/C Function Call  Tag=dsPIC_dsPIC_CFunctionCall  fctName='myPow'  INPUT_SIZE=1  INPUT1=real32  INPUT2=real32  INPUT3=--  OUTPUT_SIZE=1  OUTPUT1=real32  SampleTime=-1  InputType=[ 7 7 ]  OutputType=[ 7 ]  FctDeclaration=extern real32_T myPow(real32_T u1, real32_T u2);  FctCall=%y1 = myPow(%u1, %u2);  OrderingInOutPopup=None
  u^v : Outport
  wires:
  v/1 -> C Function Call/2
  u/1 -> C Function Call/1
  C Function Call/1 -> u^v/1

== system controlMCUSlugsMKII/Inner Loop/ Navigation/Longitudinal Channel/Compute Airspeed/Subsystem1 ==
  x : Inport
  C Function Call : dsPICdrivers/OTHERS/C Function Call  Tag=dsPIC_dsPIC_CFunctionCall  fctName='mySqrt'  INPUT_SIZE=1  INPUT1=real32  INPUT2=--  INPUT3=--  OUTPUT_SIZE=1  OUTPUT1=real32  SampleTime=-1  InputType=[ 7 ]  OutputType=[ 7 ]  FctDeclaration=extern real32_T mySqrt(real32_T u1);  FctCall=%y1 = mySqrt(%u1);  OrderingInOutPopup=None
  negprotect : Stateflow chart
  sqrt(x) : Outport
  wires:
  x/1 -> negprotect/1(val)
  negprotect/1(zpVal) -> C Function Call/1
  C Function Call/1 -> sqrt(x)/1

== system controlMCUSlugsMKII/Inner Loop/ Navigation/Navigation/Compute WP Index/Compute P ==
  WP1 : Inport  Orientation=left
  T1 : Inport  Port=2
  WP2 : Inport  Orientation=left  Port=3
  U_com : Inport  Port=4
  GS R_in : Inport  Orientation=left  Port=5
  GS LLA : Inport  Orientation=left  Port=6
  Groundspeed : Inport  Port=7
  Preturn Constant : Inport  Port=8
  Enable : EnablePort
  Add : Sum  Inputs=2  OutScaling=2^-10
  Compute R : Subsystem
  Compute T  in Frenet : Subsystem  Orientation=left  AncestorBlock=SLUGS_Library/Navigation/Compute Frenet
  Demux : Demux  Orientation=left  Outputs=3
  Geod2LTP1 : Subsystem  Orientation=left
      mask Description:
      | This block provides transformation of the Geodetic coordinates
      | to the LTP coorinate system. The block uses two consecutive transformations
      | (Geodetic -> ECEF ->LTP).
      | Geodetic coordinates of the LTP origin should also be predetermined.
      mask Help: Oops!
      mask Display: plot(0,0,100,100,[45,40,35,40,40],[85,95,85,95,40],[85,95,85,95,40],[35,40,45,40,40],[60,40,10,20,10,14],[70,40,10,13,10,20],[56,45],[70,70],[60,60],[50,60],[60,60],[30,40],[50,60],[20,20],[30,40],[20,20],[45,55],[35,25],[75,65],[35,25])
  Get Circles : Subsystem
  IC : InitialCondition  Value=50
  Integer Delay1 : simulink/Discrete/Integer Delay  vinit=0.0  samptime=-1  NumDelays=1
  Integer Delay2 : simulink/Discrete/Integer Delay  Orientation=left  vinit=0.0  samptime=-1  NumDelays=1
  Product1 : Product  OutDataTypeMode=single  RndMeth=Zero
  WP1_1 : InportShadow  Port=1  LatchByCopyingInsideSignal=off
  get WP Coord from Index : Subsystem  Orientation=left  AncestorBlock=SLUGS_Library/Navigation/get WP Coord from Index
  P : Outport  InitialOutput=50
  wires:
  IC/1 -> P/1
  GS LLA/1 -> Geod2LTP1/1(GS Lat,Lon)
  GS R_in/1 -> Geod2LTP1/2(GS ECEF)
  get WP Coord from Index/1(WP Coord) -> Demux/1
  Geod2LTP1/1("NEU, m") -> Integer Delay2/1
  Demux/3 -> Geod2LTP1/5(Hight,m(GPS))
  Demux/2 -> Geod2LTP1/4("Lon, deg(GPS)")
  Demux/1 -> Geod2LTP1/3("Lat, deg(GPS)")
  Integer Delay1/1 -> Get Circles/1(T1)
  WP1_1/1 -> Get Circles/3("Wp_to ")
  T1/1 -> Integer Delay1/1
  WP2/1 -> get WP Coord from Index/1(WP Idx)
  WP1/1 -> Compute T  in Frenet/1(Pos 1)
  Compute T  in Frenet/1(T) -> Get Circles/2(T2)
  Integer Delay2/1 -> Compute T  in Frenet/2(Pos 2)
  Compute R/1(R) -> Get Circles/4(R)
  U_com/1 -> Compute R/1(U_com)
  Product1/1 -> Add/1
  Groundspeed/1 -> Product1/2
  Preturn Constant/1 -> Product1/1
  Get Circles/1(P) -> Add/2
  Add/1 -> IC/1

== system controlMCUSlugsMKII/Inner Loop/ Navigation/Navigation/Compute WP Index/Grab IC ==
  UAV Pos : Inport
  Enable : EnablePort
  Compute GS Location : Subsystem
  Constant : Constant  Value=11  OutDataTypeMode=uint8
  Selector : Selector  IndexOptions=Index vector (dialog)  Indices=[3 1 2]  OutputSizes=1  InputPortWidth=3
  get GS Location (WP 11 is GS) : Subsystem  AncestorBlock=SLUGS_Library/Navigation/get WP Coord from Index
  IC : Outport
  "GS, Lat Lon" : Outport  Port=2
  GS R_in : Outport  Port=3
  wires:
  get GS Location (WP 11 is GS)/1(WP Coord) -> Selector/1
  Selector/1 -> Compute GS Location/1(GS Location)
  Compute GS Location/2(R_in) -> GS R_in/1
  Compute GS Location/1("Lat, Lon") -> "GS, Lat Lon"/1
  Constant/1 -> get GS Location (WP 11 is GS)/1(WP Idx)
  UAV Pos/1 -> IC/1

== system controlMCUSlugsMKII/Inner Loop/ Navigation/Navigation/Compute WP Index/Subsystem ==
  WP Fly : Inport
  Add1 : Sum  Inputs=2  OutScaling=2^-10
  Hit  Crossing1 : HitCross  HitCrossingOffset=0.3  HitCrossingDirection=rising  SampleTime=apSampleTime
  Integer Delay1 : simulink/Discrete/Integer Delay  vinit=0  samptime=-1  NumDelays=1
  Just Enab : Outport
  wires:
  WP Fly/1 -> Hit  Crossing1/1
  Add1/1 -> Just Enab/1
  Hit  Crossing1/1 -> Integer Delay1/1, Add1/2
  Integer Delay1/1 -> Add1/1

== system controlMCUSlugsMKII/Inner Loop/ Navigation/Navigation/Compute WP Index/Subsystem1 ==
  swInc : Inport  Orientation=down
  Add : Sum  Orientation=left  Inputs=2  OutScaling=2^-10
  IC : InitialCondition  Orientation=down
  Integer Delay2 : simulink/Discrete/Integer Delay  Orientation=left  vinit=0  samptime=-1  NumDelays=1
  swEna : Outport  Orientation=left
  wires:
  swInc/1 -> IC/1
  Add/1 -> swEna/1
  IC/1 -> Add/2, Integer Delay2/1
  Integer Delay2/1 -> Add/1

== system controlMCUSlugsMKII/Inner Loop/ Navigation/Navigation/Compute WP Index/Switch when  in Line Segment ==
  P : Inport
  WP0 Idx : Inport  Port=2
  Puav : Inport  Port=3
  "WP1 " : Inport  Port=4
  WP0 : Inport  Port=5
  T : Inport  Port=6
  1st WP : Switch  Criteria=u2 > Threshold  Threshold=0.3
  Compare To Zero : simulink/Logic and Bit Operations/Compare To Zero  SystemSampleTime=-1  relop=>  LogicOutDataTypeMode=uint8  ZeroCross=off
  Compute  Projection : Subsystem
  Compute Total Run : Subsystem
  IC : InitialCondition
  Integer Delay1 : simulink/Discrete/Integer Delay  vinit=0  samptime=-1  NumDelays=1
  Subsystem1 : Subsystem
  Switch Distance Less than? : RelationalOperator  LogicOutDataTypeMode=Specify via dialog  SampleTime=apSampleTime
  Switch Distance WP0 : Constant  Value=100  OutDataTypeMode=single
  WP Update : Subsystem  mask{T=0.01}
      mask prompts: T "Sample Time"
  "WP0   " : InportShadow  Port=5  LatchByCopyingInsideSignal=off
  Switch LS : Outport
  Tot Run : Outport  Port=2
  Dg : Outport  Port=3
  wires:
  Compute  Projection/1(Dg) -> Switch Distance Less than?/1, Dg/1
  Subsystem1/1(swEna) -> IC/1
  WP Update/1(Update?) -> Subsystem1/1(swInc)
  "WP0   "/1 -> WP Update/1(XYZ), Compute Total Run/2("WP0  ")
  "WP1 "/1 -> Compute Total Run/1(WP1)
  Compute Total Run/1(Tot Run) -> Switch Distance Less than?/2, Tot Run/1
  Puav/1 -> Compute  Projection/1(Puav)
  WP0/1 -> Compute  Projection/2(WP0)
  T/1 -> Compute  Projection/3(T)
  Switch Distance Less than?/1 -> Switch LS/1
  WP0 Idx/1 -> Integer Delay1/1
  P/1 -> 1st WP/1
  1st WP/1 -> Compute Total Run/3(P)
  Integer Delay1/1 -> Compare To Zero/1
  Switch Distance WP0/1 -> 1st WP/3
  Compare To Zero/1 -> 1st WP/2
  IC/1 -> Compute Total Run/Enable

== system controlMCUSlugsMKII/Inner Loop/ Navigation/Navigation/Get Wps Compute Frenet/Geod2LTP1 ==
  GS Lat,Lon : Inport
  GS ECEF : Inport  Port=2
  "Lat, deg(GPS)" : Inport  Port=3
  "Lon, deg(GPS)" : Inport  Port=4
  Hight,m(GPS) : Inport  Port=5
  ECEF2LTP (UEN) : Subsystem
      mask Display: plot(0,0,100,100,[45,40,35,40,40],[85,95,85,95,40],[85,95,85,95,40],[35,40,45,40,40],[60,40,10,20,10,14],[70,40,10,13,10,20],[56,45],[70,70],[60,60],[50,60],[60,60],[30,40],[50,60],[20,20],[30,40],[20,20],[45,55],[35,25],[75,65],[35,25])
  Geod2ECEF1 : Subsystem  mask{Re=6378137, Rp=6356752.3142}
      mask prompts: Re "Enter equatorial radius, m"; Rp "Enter polar radius,m"
  Mux : Mux  Inputs=3
  Reshape : Reshape  OutputDimensionality=Column vector (2-D)
  Reshape1 : Reshape
  Sum1 : Sum  Inputs=|+-  OutDataTypeMode=single  SaturateOnIntegerOverflow=on
  UEN 2 NEU : Gain  Gain=[0 0 1;0 1 0;1 0 0]  Multiplication=Matrix(K*u)  OutDataTypeMode=Specify via dialog  OutDataType=float('single')  SaturateOnIntegerOverflow=on
  "NEU, m" : Outport
  wires:
  UEN 2 NEU/1 -> Reshape1/1
  Geod2ECEF1/3("Ze, m ") -> Mux/3
  Geod2ECEF1/1("Xe, m ") -> Mux/1
  Geod2ECEF1/2("Ye, m ") -> Mux/2
  "Lat, deg(GPS)"/1 -> Geod2ECEF1/2("lat, deg")
  "Lon, deg(GPS)"/1 -> Geod2ECEF1/3(lon,deg)
  GS Lat,Lon/1 -> ECEF2LTP (UEN)/2("Long, Lat")
  GS ECEF/1 -> Sum1/2
  ECEF2LTP (UEN)/1(Out) -> Reshape/1  "Moving Side"
  Hight,m(GPS)/1 -> Geod2ECEF1/1("height, m")
  Mux/1 -> Sum1/1  "r_mov"
  Sum1/1 -> ECEF2LTP (UEN)/1(ECEF coordinates)
  Reshape/1 -> UEN 2 NEU/1
  Reshape1/1 -> "NEU, m"/1

== system controlMCUSlugsMKII/Inner Loop/ Navigation/Navigation/Get Wps Compute Frenet/Geod2LTP2 ==
  GS Lat,Lon : Inport
  GS ECEF : Inport  Port=2
  "Lat, deg(GPS)" : Inport  Port=3
  "Lon, deg(GPS)" : Inport  Port=4
  Hight,m(GPS) : Inport  Port=5
  ECEF2LTP (UEN) : Subsystem
      mask Display: plot(0,0,100,100,[45,40,35,40,40],[85,95,85,95,40],[85,95,85,95,40],[35,40,45,40,40],[60,40,10,20,10,14],[70,40,10,13,10,20],[56,45],[70,70],[60,60],[50,60],[60,60],[30,40],[50,60],[20,20],[30,40],[20,20],[45,55],[35,25],[75,65],[35,25])
  Geod2ECEF1 : Subsystem  mask{Re=6378137, Rp=6356752.3142}
      mask prompts: Re "Enter equatorial radius, m"; Rp "Enter polar radius,m"
  Mux : Mux  Inputs=3
  Reshape : Reshape  OutputDimensionality=Column vector (2-D)
  Reshape1 : Reshape
  Sum1 : Sum  Inputs=|+-  OutDataTypeMode=single  SaturateOnIntegerOverflow=on
  UEN 2 NEU : Gain  Gain=[0 0 1;0 1 0;1 0 0]  Multiplication=Matrix(K*u)  OutDataTypeMode=Specify via dialog  OutDataType=float('single')  SaturateOnIntegerOverflow=on
  "NEU, m" : Outport
  wires:
  UEN 2 NEU/1 -> Reshape1/1
  Geod2ECEF1/3("Ze, m ") -> Mux/3
  Geod2ECEF1/1("Xe, m ") -> Mux/1
  Geod2ECEF1/2("Ye, m ") -> Mux/2
  "Lat, deg(GPS)"/1 -> Geod2ECEF1/2("lat, deg")
  "Lon, deg(GPS)"/1 -> Geod2ECEF1/3(lon,deg)
  GS Lat,Lon/1 -> ECEF2LTP (UEN)/2("Long, Lat")
  GS ECEF/1 -> Sum1/2
  ECEF2LTP (UEN)/1(Out) -> Reshape/1  "Moving Side"
  Hight,m(GPS)/1 -> Geod2ECEF1/1("height, m")
  Mux/1 -> Sum1/1  "r_mov"
  Sum1/1 -> ECEF2LTP (UEN)/1(ECEF coordinates)
  Reshape/1 -> UEN 2 NEU/1
  Reshape1/1 -> "NEU, m"/1

== system controlMCUSlugsMKII/Inner Loop/ Navigation/Navigation/Get Wps Compute Frenet/get WP Coord from Index ==
  WP Idx : Inport
  C Function Call : dsPICdrivers/OTHERS/C Function Call  Tag=dsPIC_dsPIC_CFunctionCall  fctName='getWP'  INPUT_SIZE=1  INPUT1=uint8  INPUT2=--  INPUT3=--  OUTPUT_SIZE=3  OUTPUT1=real32  SampleTime=-1  InputType=[ 2 ]  OutputType=[ 7 ]  FctDeclaration=extern void getWP(uint8_T u1,real32_T* y1);  FctCall=getWP(%u1, *%y1);  OrderingInOutPopup=None
  WP Coord : Outport
  wires:
  WP Idx/1 -> C Function Call/1
  C Function Call/1 -> WP Coord/1

== system controlMCUSlugsMKII/Inner Loop/ Navigation/Navigation/Get Wps Compute Frenet/get WP Coord from Index  ==
  WP Idx : Inport
  C Function Call : dsPICdrivers/OTHERS/C Function Call  Tag=dsPIC_dsPIC_CFunctionCall  fctName='getWP'  INPUT_SIZE=1  INPUT1=uint8  INPUT2=--  INPUT3=--  OUTPUT_SIZE=3  OUTPUT1=real32  SampleTime=-1  InputType=[ 2 ]  OutputType=[ 7 ]  FctDeclaration=extern void getWP(uint8_T u1,real32_T* y1);  FctCall=getWP(%u1, *%y1);  OrderingInOutPopup=None
  WP Coord : Outport
  wires:
  WP Idx/1 -> C Function Call/1
  C Function Call/1 -> WP Coord/1

== system controlMCUSlugsMKII/Inner Loop/ Navigation/Navigation/Park, Deyst & How Lat Accel Cmd/Compute Eta ==
  Vxyz : Inport
  L2_vec : Inport  Port=2
  Ground Speed : Inport  Port=3
  3x3 Cross Product : aerolibutil/3x3 Cross Product  SystemSampleTime=-1
  Divide5 : Product  Inputs=*//  OutScaling=2^-10
  Norm : SLUGS_Library/Navigation/Norm  SystemSampleTime=-1
  Selector : Selector  IndexOptions=Index vector (dialog)  Indices=[3]  OutputSizes=1  InputPortWidth=3
  Subsystem6 : SLUGS_Library/Subsystem6  SystemSampleTime=-1
  To Workspace : ToWorkspace  VariableName=L1  SampleTime=-1  SaveFormat=Array
  To Workspace1 : ToWorkspace  VariableName=Vned  SampleTime=-1  SaveFormat=Array
  To Workspace2 : ToWorkspace  VariableName=eta  SampleTime=-1  SaveFormat=Array
  negprotect : Stateflow chart
  Eta : Outport
  wires:
  negprotect/1(zpVal) -> Divide5/2
  L2_vec/1 -> To Workspace/1, 3x3 Cross Product/2, Norm/1
  Divide5/1 -> Selector/1
  Norm/1 -> negprotect/1(val)
  3x3 Cross Product/1 -> Divide5/1
  Vxyz/1 -> 3x3 Cross Product/1, To Workspace1/1
  Selector/1 -> Subsystem6/1
  Subsystem6/1 -> Eta/1, To Workspace2/1
  Ground Speed/1 -> Divide5/3

== system controlMCUSlugsMKII/Inner Loop/ Navigation/Navigation/Park, Deyst & How Lat Accel Cmd/Compute L2 Vector LINE MODE ==
  Pe_lat : Inport
  L2 : Inport  Port=2
  T : Inport  Port=3
  N : Inport  Port=4
  Add : Sum  Inputs=-+  OutScaling=2^-10
  Add2 : Sum  Inputs=-+  OutScaling=2^-10
  Divide{,1..3} (4 alike) : Product  OutScaling=2^-10
  Gain : Gain  Orientation=up  Gain=-1
  Subsystem1 : SLUGS_Library/Subsystem1  SystemSampleTime=-1
  Subsystem9 : SLUGS_Library/Subsystem9  SystemSampleTime=-1
  To Workspace3 : ToWorkspace  VariableName=Pey  SampleTime=-1  SaveFormat=Array
  L2_vec : Outport
  wires:
  Divide3/1 -> Add2/2  "||CD||*T"
  T/1 -> Divide3/1
  N/1 -> Divide2/1
  Divide2/1 -> Add2/1  "N*Pey"
  Subsystem1/1 -> Divide3/2  "||CD||"
  Add/1 -> Subsystem9/1
  Divide/1 -> Add/2
  Divide1/1 -> Add/1
  Pe_lat/1 -> Divide1/1, Divide1/2, To Workspace3/1, Gain/1
  L2/1 -> Divide/2, Divide/1
  Gain/1 -> Divide2/2
  Add2/1 -> L2_vec/1  "L1_vec"
  Subsystem9/1 -> Subsystem1/1
